simulink model "rotary_pendulum_sldrt"  (R2024a)
settings: Solver=ode1  StartTime=0.0  StopTime=inf  FixedStep=Ts  RelTol=1e-3
PostLoadFcn:
  | try
  | if isempty(which('ZHAWcbfcn'));
  | callback_fid07124=fopen('ZHAWcbfcn.m','w');
  | [~]=fprintf(callback_fid07124,'%s',get_param([bdroot,'/ Setup SLDRT'],'ClipboardFcn'));
  | [~]=fclose(callback_fid07124);
  | setpref('ZHAW_SLDRT_lib','cb_fcn',which('ZHAWcbfcn'))
  | clear callback_fid07124
  | end
  | catch
  | clear callback_fid07124
  | end
  | Ts=eval(get_param([bdroot,'/ Setup SLDRT'],'Ts'));
InitFcn:
  | Ts=eval(get_param([bdroot,'/ Setup SLDRT'],'Ts'));
undefined symbols (not defined in the file): i_max, Kp_i, Kp_om, National_Instruments, PCIe, phi2_disable, phi2_enable, Tn_i, Tn_om, u_max
libraries: sldrtlib x5, cstblocks x2, simulink x1
(part 2 of 2)

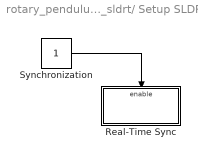
== system rotary_pendulum_sldrt/ Setup SLDRT ==
  Real-Time Sync : Subsystem
  Synchronization : Constant
  wires:
  Synchronization/1 -> Real-Time Sync/Enable

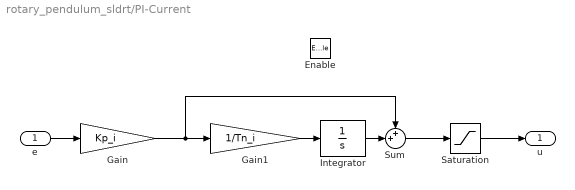
== system rotary_pendulum_sldrt/PI-Current ==
  e : Inport
  Enable : EnablePort  StatesWhenEnabling=reset
  Gain : Gain  Gain=Kp_i
  Gain1 : Gain  Gain=1/Tn_i
  Integrator : Integrator  LimitOutput=on  UpperSaturationLimit=u_max  LowerSaturationLimit=-u_max
  Saturation : Saturate  UpperLimit=u_max  LowerLimit=-u_max
  Sum : Sum  Inputs=++|
  u : Outport  OutputWhenDisabled=reset  InitialOutput=0
  wires:
  Gain/1 -> Gain1/1, Sum/1
  Saturation/1 -> u/1
  Sum/1 -> Saturation/1
  Integrator/1 -> Sum/2
  Gain1/1 -> Integrator/1
  e/1 -> Gain/1

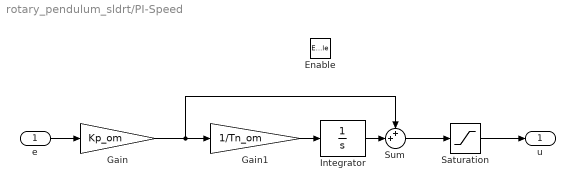
== system rotary_pendulum_sldrt/PI-Speed ==
  e : Inport
  Enable : EnablePort  StatesWhenEnabling=reset
  Gain : Gain  Gain=Kp_om
  Gain1 : Gain  Gain=1/Tn_om
  Integrator : Integrator  LimitOutput=on  UpperSaturationLimit=i_max  LowerSaturationLimit=-i_max
  Saturation : Saturate  UpperLimit=i_max  LowerLimit=-i_max
  Sum : Sum  Inputs=++|
  u : Outport  OutputWhenDisabled=reset  InitialOutput=0
  wires:
  e/1 -> Gain/1
  Gain1/1 -> Integrator/1
  Integrator/1 -> Sum/2
  Sum/1 -> Saturation/1
  Saturation/1 -> u/1
  Gain/1 -> Sum/1, Gain1/1

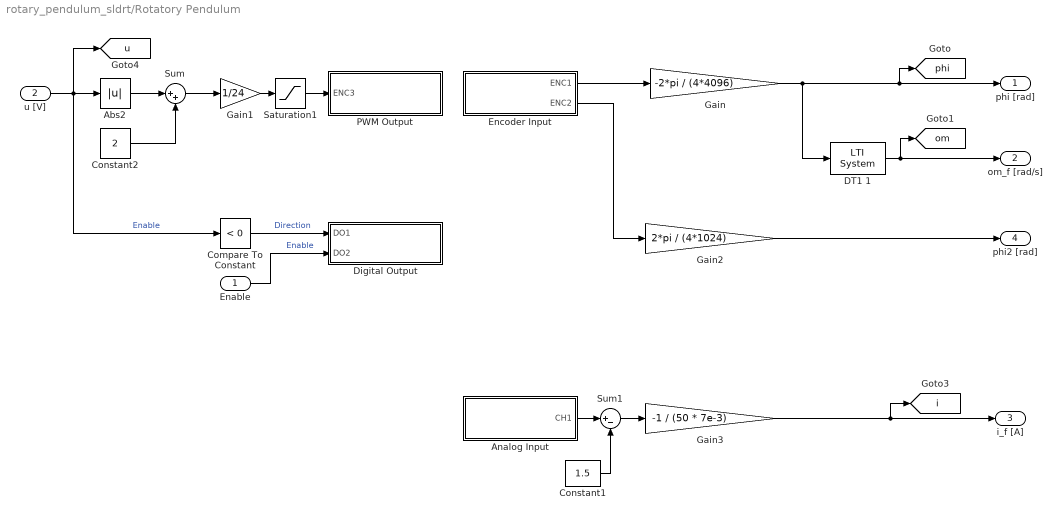
== system rotary_pendulum_sldrt/Rotatory Pendulum ==
  Enable : Inport
  u [V] : Inport  Port=2
  Abs2 : Abs  SaturateOnIntegerOverflow=off
  Analog Input : Subsystem  mask(NI Analog Input){device=PCIe-6321, connect=Banana Terminal, couple=differential, ch1=on, ch9=off, ch2=off, ch10=off, ch3=off, ch11=off, ch4=off, ch12=off, ch5=off, ch13=off, ch6=off, ch14=off, ch7=off, ch15=off, ch8=off, ch16=off, Ts=Ts}
      mask prompts: device "NI Device Type:"; connect "Connector Box:"; couple "CH Coupling:"; ch1 "CH1-CH9"; ch9 "CH9-GND"; ch2 "CH2-CH10"; ch10 "CH10-GND"; ch3 "CH3-CH11"; ch11 "CH11-GND"; ch4 "CH4-CH12"; ch12 "CH12-GND"; ch5 "CH5-CH13"; ch13 "CH13-GND"; ch6 "CH6-CH14"; ch14 "CH14-GND"; ch7 "CH7-CH15"; ch15 "CH15-GND"; ch8 "CH8-CH16"; ch16 "CH16-GND"; Ts "Sample Time:"
      mask help:
      | AD Converter
      | +/-10V
      mask init:
      | try ch_list = ZHAWcbfcn('get_ch_list'); end
      | try ZHAWcbfcn('BlockUpdate'); end
      settings: AttributesFormatString=%<couple>  OpenFcn=try ZHAWcbfcn('openMask'); end
      settings: CopyFcn=|
      | try
      | ZHAWcbfcn('CopyIOblock')
      | end
      | set_param(gcb,'OpenFcn','try ZHAWcbfcn(''openMask''); end')
      mask TypeOptions device: PCI-6221 | PCI-6259 | PCIe-6259 | PCIe-6321 | PCIe-6363
      mask TypeOptions connect: BNC Terminal | Banana Terminal | Screw Terminal
      mask Callback connect:
      | try ZHAWcbfcn('SetConnectorBox'); end
      | try ZHAWcbfcn('SetChannelCoupling'); end
      mask TypeOptions couple: single ended | differential
      mask Callback couple:
      | try ZHAWcbfcn('SetChannelCoupling'); end
      | try ZHAWcbfcn('SetConnectorBox'); end
      mask DialogControl DescGroupVar Prompt: NI Analog Input (R2024a)
      mask Display: disp('NI\nPCIe-6321')
  Compare To Constant : simulink/Logic and Bit Operations/Compare To Constant  relop=<  const=0  OutDataTypeStr=boolean
  Constant1 : Constant  Value=1.5
  Constant2 : Constant  Value=2
  DT1 1 : cstblocks/LTI System  sys=G_phi2omf  IC=[]  PadeOrder=0
  Digital Output : Subsystem  mask(NI Digital Output){device=PCIe-6321, connect=Banana Terminal, ch1=on, ch2=on, ch3=off, ch4=off, ch5=off, ch6=off, ch7=off, ch8=off, Ts=Ts}
      mask prompts: device "NI Device Type:"; connect "Connector Box:"; ch1 "DO1"; ch2 "DO2"; ch3 "DO3"; ch4 "DO4"; ch5 "DO5"; ch6 "DO6"; ch7 "DO7"; ch8 "DO8"; Ts "Sample Time:"
      mask help: Digital output 5V TTL.
      mask init:
      | try ch_list = ZHAWcbfcn('get_ch_list'); end
      | try ZHAWcbfcn('BlockUpdate'); end
      settings: OpenFcn=try ZHAWcbfcn('openMask'); end
      settings: CopyFcn=|
      | try
      | ZHAWcbfcn('CopyIOblock')
      | end
      | set_param(gcb,'OpenFcn','try ZHAWcbfcn(''openMask''); end')
      mask TypeOptions device: PCI-6221 | PCI-6259 | PCIe-6259 | PCIe-6321 | PCIe-6363
      mask Callback device: try ZHAWcbfcn('SetChannelNumber'); end
      mask TypeOptions connect: BNC Terminal | Banana Terminal | Screw Terminal
      mask Callback connect: try ZHAWcbfcn('SetConnectorBox'); end
      mask DialogControl DescGroupVar Prompt: NI Digital Output (R2024a)
      mask Display: disp('NI\nPCIe-6321')
  Encoder Input : Subsystem  mask(NI Encoder Input){device=PCIe-6321, connect=Banana Terminal, reset=off, ch1=on, ch2=on, ch3=off, ch4=off, Ts=Ts}
      mask prompts: device "NI Device Type:"; connect "Connector Box:"; reset "Reset at Index:"; ch1 "ENC1"; ch2 "ENC2"; ch3 "ENC3"; ch4 "ENC4"; Ts "Sample Time:"
      mask help:
      | Quadratur Encoder.
      | X4 Decoding.
      | Output is increments.
      mask init:
      | try ch_list = ZHAWcbfcn('get_ch_list'); end
      | try ZHAWcbfcn('BlockUpdate'); end
      settings: AttributesFormatString=Index Reset: %<reset>  OpenFcn=try ZHAWcbfcn('openMask'); end
      settings: CopyFcn=|
      | try
      | ZHAWcbfcn('CopyIOblock')
      | end
      | set_param(gcb,'OpenFcn','try ZHAWcbfcn(''openMask''); end')
      mask TypeOptions device: PCI-6221 | PCI-6259 | PCIe-6259 | PCIe-6321 | PCIe-6363
      mask Callback device: try ZHAWcbfcn('SetChannelNumber'); end
      mask TypeOptions connect: BNC Terminal | Banana Terminal | Screw Terminal
      mask Callback connect: try ZHAWcbfcn('SetConnectorBox'); end
      mask TypeOptions reset: on | off
      mask Callback reset: try ZHAWcbfcn('SetEncoderReset'); end
      mask DialogControl DescGroupVar Prompt: NI Encoder Input (R2024a)
      mask Display: disp('NI\nPCIe-6321')
  Gain : Gain  Gain=-2*pi / (4*4096)
  Gain1 : Gain  Gain=1/24
  Gain2 : Gain  Gain=2*pi / (4*1024)
  Gain3 : Gain  Gain=-1 / (50 * 7e-3)
  PWM Output : Subsystem  mask(NI PWM Output){device=PCIe-6321, connect=Banana Terminal, mode=PWM, ch1=off, ch2=off, ch3=on, ch4=off, pwm_frequ=20e3, duty=0, Ts_copy=Ts}
      mask prompts: device "NI Device Type:"; connect "Connector Box :"; mode "Output Modus:"; ch1 "ENC1"; ch2 "ENC2"; ch3 "ENC3"; ch4 "ENC4"; pwm_frequ "PWM Frequency [Hz]:"; duty "Duty Cycle [0...1]:"; Ts_copy "Sample Time:"
      mask help:
      | PWM or Frequency output.
      |
      | PWM:
      | The input specifies the duty cycle as a decimal fraction from 0 through 1 inclusive.
      | It determines the amount of time that the output signal value is high (1).
      |
      | Frequency;
      | The input specifies the output frequency in [Hz].
      mask init:
      | try ch_list = ZHAWcbfcn('get_ch_list'); end
      | try ZHAWcbfcn('BlockUpdate'); end
      settings: OpenFcn=try ZHAWcbfcn('openMask'); end
      settings: CopyFcn=|
      | try
      | ZHAWcbfcn('CopyIOblock')
      | end
      | set_param(gcb,'OpenFcn','try ZHAWcbfcn(''openMask''); end')
      mask TypeOptions device: PCI-6221 | PCI-6259 | PCIe-6259 | PCIe-6321 | PCIe-6363
      mask Callback device: try ZHAWcbfcn('SetChannelNumber'); end
      mask TypeOptions connect: BNC Terminal | Banana Terminal | Screw Terminal
      mask Callback connect: try ZHAWcbfcn('SetConnectorBox'); end
      mask TypeOptions mode: PWM | Frequency
      mask DialogControl DescGroupVar Prompt: NI Analog Output (R2024a)
      mask Display: disp('NI\nPCIe-6321')
  Saturation1 : Saturate  UpperLimit=1  LowerLimit=0
  Sum : Sum  Inputs=|++
  Sum1 : Sum  Inputs=|+-
  phi [rad] : Outport
  om_f [rad/s] : Outport  Port=2
  i_f [A] : Outport  Port=3
  phi2 [rad] : Outport  Port=4
  tag scope: i=global, om=global, phi=global, u=global
  wires:
  Compare To Constant/1 -> Digital Output/1(DO1)  "Direction"
  Gain/1 -> [phi], phi [rad]/1, DT1 1/1
  Encoder Input/1(ENC1) -> Gain/1
  u [V]/1 -> Compare To Constant/1, Abs2/1, [u]  "Enable"
  Enable/1 -> Digital Output/2(DO2)  "Enable"
  Analog Input/1(CH1) -> Sum1/1
  Constant1/1 -> Sum1/2
  Sum1/1 -> Gain3/1
  Gain3/1 -> [i], i_f [A]/1
  DT1 1/1 -> [om], om_f [rad/s]/1
  Saturation1/1 -> PWM Output/1(ENC3)
  Abs2/1 -> Sum/1
  Sum/1 -> Gain1/1
  Constant2/1 -> Sum/2
  Gain1/1 -> Saturation1/1
  Encoder Input/2(ENC2) -> Gain2/1
  Gain2/1 -> phi2 [rad]/1

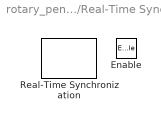
== system rotary_pendulum_sldrt/ Setup SLDRT/Real-Time Sync ==
  Enable : EnablePort
  Real-Time Synchronization : sldrtlib/Real-Time Synchronization  SampleTime=Ts  MaxMissedTicks=inf  ShowMissedTicks=off  YieldWhenWaiting=off

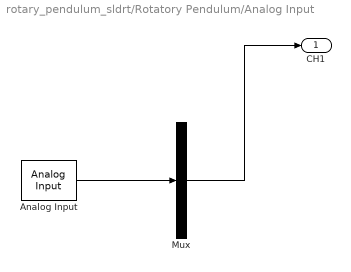
== system rotary_pendulum_sldrt/Rotatory Pendulum/Analog Input ==
  Analog Input : sldrtlib/Analog Input  SampleTime=Ts  MaxMissedTicks=10  ShowMissedTicks=off  YieldWhenWaiting=off  DrvName=National_Instruments/PCIe-6321  DrvAddress=4294967295  DrvOptions="[1  3  0  2  2  3  2]"  Channels=ch_list  RangeMode=1  VoltRange=1  DataType=1
      settings: AttributesFormatString=National Instruments\nPCIe-6321 [auto]
  Mux : Demux  Outputs=1
  CH1 : Outport  VectorParamsAs1DForOutWhenUnconnected=off
  wires:
  Mux/1 -> CH1/1
  Analog Input/1 -> Mux/1

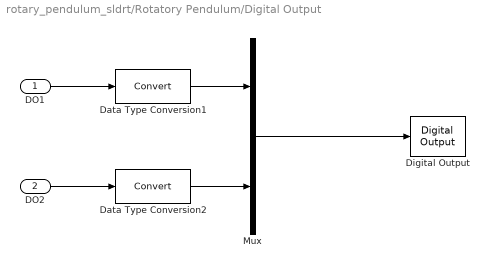
== system rotary_pendulum_sldrt/Rotatory Pendulum/Digital Output ==
  DO1 : Inport
  DO2 : Inport  Port=2
  Data Type Conversion1 : DataTypeConversion  SaturateOnIntegerOverflow=off  RndMeth=Floor
  Data Type Conversion2 : DataTypeConversion  SaturateOnIntegerOverflow=off  RndMeth=Floor
  Digital Output : sldrtlib/Digital Output  SampleTime=Ts  MaxMissedTicks=10  ShowMissedTicks=off  YieldWhenWaiting=off  DrvName=National_Instruments/PCIe-6321  DrvAddress=4294967295  DrvOptions="[1  3  0  2  2  3  2]"  Channels=ch_list  BitMode=1  InitialValue=0  FinalValue=0
      settings: AttributesFormatString=National Instruments\nPCIe-6321 [auto]
  Mux : Mux  Inputs=2
  wires:
  DO1/1 -> Data Type Conversion1/1
  DO2/1 -> Data Type Conversion2/1
  Mux/1 -> Digital Output/1
  Data Type Conversion1/1 -> Mux/1
  Data Type Conversion2/1 -> Mux/2

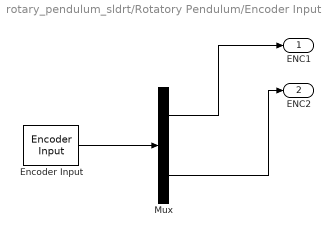
== system rotary_pendulum_sldrt/Rotatory Pendulum/Encoder Input ==
  Encoder Input : sldrtlib/Encoder Input  SampleTime=Ts  MaxMissedTicks=10  ShowMissedTicks=off  YieldWhenWaiting=off  DrvName=National_Instruments/PCIe-6321  DrvAddress=4294967295  DrvOptions="[1  3  0  2  2  3  2]"  Channels=ch_list  QuadMode=3  IndexPulse=1  InputFilter=Inf  DataType=1
      settings: AttributesFormatString=National Instruments\nPCIe-6321 [auto]
  Mux : Demux  Outputs=2
  ENC1 : Outport  VectorParamsAs1DForOutWhenUnconnected=off
  ENC2 : Outport  Port=2
  wires:
  Encoder Input/1 -> Mux/1
  Mux/1 -> ENC1/1
  Mux/2 -> ENC2/1

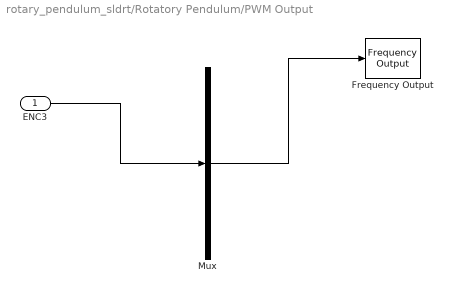
== system rotary_pendulum_sldrt/Rotatory Pendulum/PWM Output ==
  ENC3 : Inport
  Frequency Output : sldrtlib/Frequency Output  SampleTime=Ts  MaxMissedTicks=10  ShowMissedTicks=off  YieldWhenWaiting=off  DrvName=National_Instruments/PCIe-6321  DrvAddress=4294967295  DrvOptions="[1  3  0  2  2  3  2]"  Channels=ch_list  FrequencySource=1  Frequency=20e3  FrequencyFinalValue=20e3  DutySource=2  Duty=0  DutyFinalValue=0
      settings: AttributesFormatString=National Instruments\nPCIe-6321 [auto]
  Mux : Mux  Inputs=1
  wires:
  Mux/1 -> Frequency Output/1
  ENC3/1 -> Mux/1

== matlab function rotary_pendulum_sldrt/Enable in Bounds Once ==
  settings: updateMethod=DISCRETE  sampleTime=Ts
  data: phi2 input; Enable output; phi2_enable parameter; phi2_disable parameter
function Enable = fcn(phi2, phi2_enable, phi2_disable)
% One-shot hysteresis switch:
%  - Activates when   |phi2| <= phi2_enable   (only if never activated before)
%  - Deactivates when |phi2| >= phi2_disable  (after activation)
%  - Cannot be activated again once deactivated
%
% Inputs:
%   phi2         current angle in radians
%   phi2_enable  activation threshold (inner) in radians
%   phi2_disable deactivation threshold (outer) in radians
%
% Output:
%   Enable = 1 when active, 0 when inactive (locked after first deactivate)

    persistent active_state has_been_enabled_once
    if isempty(active_state)
        active_state = false;
        has_been_enabled_once = false;
    end

    % Normalize thresholds: ensure inner <= outer (bulletproofing #1)
    if phi2_disable < phi2_enable
        tmp = phi2_enable;
        phi2_enable = phi2_disable;
        phi2_disable = tmp;
    end

    if ~has_been_enabled_once
        % Enable once when inside the inner band (bulletproofing #2: inclusive)
        if abs(phi2) <= phi2_enable
            active_state = true;

        % After activation, disable once when outside the outer band (inclusive)
        elseif active_state && abs(phi2) >= phi2_disable
            active_state = false;
            has_been_enabled_once = true;   % lock out reactivation
        end
    end

    Enable = double(active_state);
end
